simulink model "ieee30"  (R2017a)
settings: Solver=VariableStepDiscrete  StartTime=0.0  StopTime=0.012  MaxStep=1e-4  RelTol=1e-3
undefined symbols (not defined in the file): Angle, Magnitude
libraries: powerlib x548
(part 4 of 4)

== system ieee30/Line 16-17-2 ==
  Line{,1..4} (5 alike) : powerlib/Elements/Three-Phase PI Section Line  LConnTagsString=a|b|c  RConnTagsString=A|B|C  Frequency=60  Resistances=[rt ro] /100  Inductances=[ lt lo] /100  Capacitances=[ct co]/100  Length=20
      settings: SourceProductName=Simscape Power Systems
  A : PMIOPort  Port=1  Side=Left
  B : PMIOPort  Port=2  Side=Left
  C : PMIOPort  Port=3  Side=Left
  a : PMIOPort  Port=4  Side=Right
  b : PMIOPort  Port=5  Side=Right
  c : PMIOPort  Port=6  Side=Right
  connections:
  Line3/RConn3 -- Line4/LConn3
  Line/RConn3 -- Line1/LConn3
  Line2/RConn3 -- Line3/LConn3
  Line2/RConn1 -- Line3/LConn1
  Line1/RConn3 -- Line2/LConn3
  Line/RConn2 -- Line1/LConn2
  Line2/RConn2 -- Line3/LConn2
  Line1/RConn1 -- Line2/LConn1
  Line3/RConn1 -- Line4/LConn1
  Line3/RConn2 -- Line4/LConn2
  Line1/RConn2 -- Line2/LConn2
  Line/RConn1 -- Line1/LConn1
  C/RConn1 -- Line/LConn3
  Line/LConn1 -- A/RConn1
  c/RConn1 -- Line4/RConn3
  a/RConn1 -- Line4/RConn1
  B/RConn1 -- Line/LConn2
  b/RConn1 -- Line4/RConn2

== system ieee30/Line 18-19-1 ==
  Line{,1..4} (5 alike) : powerlib/Elements/Three-Phase PI Section Line  LConnTagsString=a|b|c  RConnTagsString=A|B|C  Frequency=60  Resistances=[rt ro] /100  Inductances=[ lt lo] /100  Capacitances=[ct co]/100  Length=20
      settings: SourceProductName=Simscape Power Systems
  A : PMIOPort  Port=1  Side=Left
  B : PMIOPort  Port=2  Side=Left
  C : PMIOPort  Port=3  Side=Left
  a : PMIOPort  Port=4  Side=Right
  b : PMIOPort  Port=5  Side=Right
  c : PMIOPort  Port=6  Side=Right
  connections:
  Line3/RConn3 -- Line4/LConn3
  Line/RConn3 -- Line1/LConn3
  Line2/RConn3 -- Line3/LConn3
  Line2/RConn1 -- Line3/LConn1
  Line1/RConn3 -- Line2/LConn3
  Line/RConn2 -- Line1/LConn2
  Line2/RConn2 -- Line3/LConn2
  Line1/RConn1 -- Line2/LConn1
  Line3/RConn1 -- Line4/LConn1
  Line3/RConn2 -- Line4/LConn2
  Line1/RConn2 -- Line2/LConn2
  Line/RConn1 -- Line1/LConn1
  C/RConn1 -- Line/LConn3
  Line/LConn1 -- A/RConn1
  c/RConn1 -- Line4/RConn3
  a/RConn1 -- Line4/RConn1
  B/RConn1 -- Line/LConn2
  b/RConn1 -- Line4/RConn2

== system ieee30/Line 18-19-2 ==
  Line{,1..4} (5 alike) : powerlib/Elements/Three-Phase PI Section Line  LConnTagsString=a|b|c  RConnTagsString=A|B|C  Frequency=60  Resistances=[rt ro] /100  Inductances=[ lt lo] /100  Capacitances=[ct co]/100  Length=20
      settings: SourceProductName=Simscape Power Systems
  A : PMIOPort  Port=1  Side=Left
  B : PMIOPort  Port=2  Side=Left
  C : PMIOPort  Port=3  Side=Left
  a : PMIOPort  Port=4  Side=Right
  b : PMIOPort  Port=5  Side=Right
  c : PMIOPort  Port=6  Side=Right
  connections:
  Line3/RConn3 -- Line4/LConn3
  Line/RConn3 -- Line1/LConn3
  Line2/RConn3 -- Line3/LConn3
  Line2/RConn1 -- Line3/LConn1
  Line1/RConn3 -- Line2/LConn3
  Line/RConn2 -- Line1/LConn2
  Line2/RConn2 -- Line3/LConn2
  Line1/RConn1 -- Line2/LConn1
  Line3/RConn1 -- Line4/LConn1
  Line3/RConn2 -- Line4/LConn2
  Line1/RConn2 -- Line2/LConn2
  Line/RConn1 -- Line1/LConn1
  C/RConn1 -- Line/LConn3
  Line/LConn1 -- A/RConn1
  c/RConn1 -- Line4/RConn3
  a/RConn1 -- Line4/RConn1
  B/RConn1 -- Line/LConn2
  b/RConn1 -- Line4/RConn2

== system ieee30/Line 19-20-1 ==
  Line{,1..4} (5 alike) : powerlib/Elements/Three-Phase PI Section Line  LConnTagsString=a|b|c  RConnTagsString=A|B|C  Frequency=60  Resistances=[rt ro] /100  Inductances=[ lt lo] /100  Capacitances=[ct co]/100  Length=20
      settings: SourceProductName=Simscape Power Systems
  A : PMIOPort  Port=1  Side=Left
  B : PMIOPort  Port=2  Side=Left
  C : PMIOPort  Port=3  Side=Left
  a : PMIOPort  Port=4  Side=Right
  b : PMIOPort  Port=5  Side=Right
  c : PMIOPort  Port=6  Side=Right
  connections:
  Line3/RConn3 -- Line4/LConn3
  Line/RConn3 -- Line1/LConn3
  Line2/RConn3 -- Line3/LConn3
  Line2/RConn1 -- Line3/LConn1
  Line1/RConn3 -- Line2/LConn3
  Line/RConn2 -- Line1/LConn2
  Line2/RConn2 -- Line3/LConn2
  Line1/RConn1 -- Line2/LConn1
  Line3/RConn1 -- Line4/LConn1
  Line3/RConn2 -- Line4/LConn2
  Line1/RConn2 -- Line2/LConn2
  Line/RConn1 -- Line1/LConn1
  C/RConn1 -- Line/LConn3
  Line/LConn1 -- A/RConn1
  c/RConn1 -- Line4/RConn3
  a/RConn1 -- Line4/RConn1
  B/RConn1 -- Line/LConn2
  b/RConn1 -- Line4/RConn2

== system ieee30/Line 19-20-2 ==
  Line{,1..4} (5 alike) : powerlib/Elements/Three-Phase PI Section Line  LConnTagsString=a|b|c  RConnTagsString=A|B|C  Frequency=60  Resistances=[rt ro] /100  Inductances=[ lt lo] /100  Capacitances=[ct co]/100  Length=20
      settings: SourceProductName=Simscape Power Systems
  A : PMIOPort  Port=1  Side=Left
  B : PMIOPort  Port=2  Side=Left
  C : PMIOPort  Port=3  Side=Left
  a : PMIOPort  Port=4  Side=Right
  b : PMIOPort  Port=5  Side=Right
  c : PMIOPort  Port=6  Side=Right
  connections:
  Line3/RConn3 -- Line4/LConn3
  Line/RConn3 -- Line1/LConn3
  Line2/RConn3 -- Line3/LConn3
  Line2/RConn1 -- Line3/LConn1
  Line1/RConn3 -- Line2/LConn3
  Line/RConn2 -- Line1/LConn2
  Line2/RConn2 -- Line3/LConn2
  Line1/RConn1 -- Line2/LConn1
  Line3/RConn1 -- Line4/LConn1
  Line3/RConn2 -- Line4/LConn2
  Line1/RConn2 -- Line2/LConn2
  Line/RConn1 -- Line1/LConn1
  C/RConn1 -- Line/LConn3
  Line/LConn1 -- A/RConn1
  c/RConn1 -- Line4/RConn3
  a/RConn1 -- Line4/RConn1
  B/RConn1 -- Line/LConn2
  b/RConn1 -- Line4/RConn2

== system ieee30/Line 2-4-1 ==
  Line{,1..4} (5 alike) : powerlib/Elements/Three-Phase PI Section Line  LConnTagsString=a|b|c  RConnTagsString=A|B|C  Frequency=60  Resistances=[rt ro] /100  Inductances=[ lt lo] /100  Capacitances=[ct co]/100  Length=20
      settings: SourceProductName=Simscape Power Systems
  A : PMIOPort  Port=1  Side=Left
  B : PMIOPort  Port=2  Side=Left
  C : PMIOPort  Port=3  Side=Left
  a : PMIOPort  Port=4  Side=Right
  b : PMIOPort  Port=5  Side=Right
  c : PMIOPort  Port=6  Side=Right
  connections:
  Line3/RConn3 -- Line4/LConn3
  Line/RConn3 -- Line1/LConn3
  Line2/RConn3 -- Line3/LConn3
  Line2/RConn1 -- Line3/LConn1
  Line1/RConn3 -- Line2/LConn3
  Line/RConn2 -- Line1/LConn2
  Line2/RConn2 -- Line3/LConn2
  Line1/RConn1 -- Line2/LConn1
  Line3/RConn1 -- Line4/LConn1
  Line3/RConn2 -- Line4/LConn2
  Line1/RConn2 -- Line2/LConn2
  Line/RConn1 -- Line1/LConn1
  C/RConn1 -- Line/LConn3
  Line/LConn1 -- A/RConn1
  c/RConn1 -- Line4/RConn3
  a/RConn1 -- Line4/RConn1
  B/RConn1 -- Line/LConn2
  b/RConn1 -- Line4/RConn2

== system ieee30/Line 2-4-2 ==
  Line{,1..4} (5 alike) : powerlib/Elements/Three-Phase PI Section Line  LConnTagsString=a|b|c  RConnTagsString=A|B|C  Frequency=60  Resistances=[rt ro] /100  Inductances=[ lt lo] /100  Capacitances=[ct co]/100  Length=20
      settings: SourceProductName=Simscape Power Systems
  A : PMIOPort  Port=1  Side=Left
  B : PMIOPort  Port=2  Side=Left
  C : PMIOPort  Port=3  Side=Left
  a : PMIOPort  Port=4  Side=Right
  b : PMIOPort  Port=5  Side=Right
  c : PMIOPort  Port=6  Side=Right
  connections:
  Line3/RConn3 -- Line4/LConn3
  Line/RConn3 -- Line1/LConn3
  Line2/RConn3 -- Line3/LConn3
  Line2/RConn1 -- Line3/LConn1
  Line1/RConn3 -- Line2/LConn3
  Line/RConn2 -- Line1/LConn2
  Line2/RConn2 -- Line3/LConn2
  Line1/RConn1 -- Line2/LConn1
  Line3/RConn1 -- Line4/LConn1
  Line3/RConn2 -- Line4/LConn2
  Line1/RConn2 -- Line2/LConn2
  Line/RConn1 -- Line1/LConn1
  C/RConn1 -- Line/LConn3
  Line/LConn1 -- A/RConn1
  c/RConn1 -- Line4/RConn3
  a/RConn1 -- Line4/RConn1
  B/RConn1 -- Line/LConn2
  b/RConn1 -- Line4/RConn2

== system ieee30/Line 2-5-1 ==
  Line{,1..4} (5 alike) : powerlib/Elements/Three-Phase PI Section Line  LConnTagsString=a|b|c  RConnTagsString=A|B|C  Frequency=60  Resistances=[rt ro] /100  Inductances=[ lt lo] /100  Capacitances=[ct co]/100  Length=20
      settings: SourceProductName=Simscape Power Systems
  A : PMIOPort  Port=1  Side=Left
  B : PMIOPort  Port=2  Side=Left
  C : PMIOPort  Port=3  Side=Left
  a : PMIOPort  Port=4  Side=Right
  b : PMIOPort  Port=5  Side=Right
  c : PMIOPort  Port=6  Side=Right
  connections:
  Line3/RConn3 -- Line4/LConn3
  Line/RConn3 -- Line1/LConn3
  Line2/RConn3 -- Line3/LConn3
  Line2/RConn1 -- Line3/LConn1
  Line1/RConn3 -- Line2/LConn3
  Line/RConn2 -- Line1/LConn2
  Line2/RConn2 -- Line3/LConn2
  Line1/RConn1 -- Line2/LConn1
  Line3/RConn1 -- Line4/LConn1
  Line3/RConn2 -- Line4/LConn2
  Line1/RConn2 -- Line2/LConn2
  Line/RConn1 -- Line1/LConn1
  C/RConn1 -- Line/LConn3
  Line/LConn1 -- A/RConn1
  c/RConn1 -- Line4/RConn3
  a/RConn1 -- Line4/RConn1
  B/RConn1 -- Line/LConn2
  b/RConn1 -- Line4/RConn2

== system ieee30/Line 2-5-2 ==
  Line{,1..4} (5 alike) : powerlib/Elements/Three-Phase PI Section Line  LConnTagsString=a|b|c  RConnTagsString=A|B|C  Frequency=60  Resistances=[rt ro] /100  Inductances=[ lt lo] /100  Capacitances=[ct co]/100  Length=20
      settings: SourceProductName=Simscape Power Systems
  A : PMIOPort  Port=1  Side=Left
  B : PMIOPort  Port=2  Side=Left
  C : PMIOPort  Port=3  Side=Left
  a : PMIOPort  Port=4  Side=Right
  b : PMIOPort  Port=5  Side=Right
  c : PMIOPort  Port=6  Side=Right
  connections:
  Line3/RConn3 -- Line4/LConn3
  Line/RConn3 -- Line1/LConn3
  Line2/RConn3 -- Line3/LConn3
  Line2/RConn1 -- Line3/LConn1
  Line1/RConn3 -- Line2/LConn3
  Line/RConn2 -- Line1/LConn2
  Line2/RConn2 -- Line3/LConn2
  Line1/RConn1 -- Line2/LConn1
  Line3/RConn1 -- Line4/LConn1
  Line3/RConn2 -- Line4/LConn2
  Line1/RConn2 -- Line2/LConn2
  Line/RConn1 -- Line1/LConn1
  C/RConn1 -- Line/LConn3
  Line/LConn1 -- A/RConn1
  c/RConn1 -- Line4/RConn3
  a/RConn1 -- Line4/RConn1
  B/RConn1 -- Line/LConn2
  b/RConn1 -- Line4/RConn2

== system ieee30/Line 2-6-1 ==
  Line{,1..4} (5 alike) : powerlib/Elements/Three-Phase PI Section Line  LConnTagsString=a|b|c  RConnTagsString=A|B|C  Frequency=60  Resistances=[rt ro] /100  Inductances=[ lt lo] /100  Capacitances=[ct co]/100  Length=20
      settings: SourceProductName=Simscape Power Systems
  A : PMIOPort  Port=1  Side=Left
  B : PMIOPort  Port=2  Side=Left
  C : PMIOPort  Port=3  Side=Left
  a : PMIOPort  Port=4  Side=Right
  b : PMIOPort  Port=5  Side=Right
  c : PMIOPort  Port=6  Side=Right
  connections:
  Line3/RConn3 -- Line4/LConn3
  Line/RConn3 -- Line1/LConn3
  Line2/RConn3 -- Line3/LConn3
  Line2/RConn1 -- Line3/LConn1
  Line1/RConn3 -- Line2/LConn3
  Line/RConn2 -- Line1/LConn2
  Line2/RConn2 -- Line3/LConn2
  Line1/RConn1 -- Line2/LConn1
  Line3/RConn1 -- Line4/LConn1
  Line3/RConn2 -- Line4/LConn2
  Line1/RConn2 -- Line2/LConn2
  Line/RConn1 -- Line1/LConn1
  C/RConn1 -- Line/LConn3
  Line/LConn1 -- A/RConn1
  c/RConn1 -- Line4/RConn3
  a/RConn1 -- Line4/RConn1
  B/RConn1 -- Line/LConn2
  b/RConn1 -- Line4/RConn2

== system ieee30/Line 2-6-2 ==
  Line{,1..4} (5 alike) : powerlib/Elements/Three-Phase PI Section Line  LConnTagsString=a|b|c  RConnTagsString=A|B|C  Frequency=60  Resistances=[rt ro] /100  Inductances=[ lt lo] /100  Capacitances=[ct co]/100  Length=20
      settings: SourceProductName=Simscape Power Systems
  A : PMIOPort  Port=1  Side=Left
  B : PMIOPort  Port=2  Side=Left
  C : PMIOPort  Port=3  Side=Left
  a : PMIOPort  Port=4  Side=Right
  b : PMIOPort  Port=5  Side=Right
  c : PMIOPort  Port=6  Side=Right
  connections:
  Line3/RConn3 -- Line4/LConn3
  Line/RConn3 -- Line1/LConn3
  Line2/RConn3 -- Line3/LConn3
  Line2/RConn1 -- Line3/LConn1
  Line1/RConn3 -- Line2/LConn3
  Line/RConn2 -- Line1/LConn2
  Line2/RConn2 -- Line3/LConn2
  Line1/RConn1 -- Line2/LConn1
  Line3/RConn1 -- Line4/LConn1
  Line3/RConn2 -- Line4/LConn2
  Line1/RConn2 -- Line2/LConn2
  Line/RConn1 -- Line1/LConn1
  C/RConn1 -- Line/LConn3
  Line/LConn1 -- A/RConn1
  c/RConn1 -- Line4/RConn3
  a/RConn1 -- Line4/RConn1
  B/RConn1 -- Line/LConn2
  b/RConn1 -- Line4/RConn2

== system ieee30/Line 21-22-1 ==
  Line{,1..4} (5 alike) : powerlib/Elements/Three-Phase PI Section Line  LConnTagsString=a|b|c  RConnTagsString=A|B|C  Frequency=60  Resistances=[rt ro] /100  Inductances=[ lt lo] /100  Capacitances=[ct co]/100  Length=20
      settings: SourceProductName=Simscape Power Systems
  A : PMIOPort  Port=1  Side=Left
  B : PMIOPort  Port=2  Side=Left
  C : PMIOPort  Port=3  Side=Left
  a : PMIOPort  Port=4  Side=Right
  b : PMIOPort  Port=5  Side=Right
  c : PMIOPort  Port=6  Side=Right
  connections:
  Line3/RConn3 -- Line4/LConn3
  Line/RConn3 -- Line1/LConn3
  Line2/RConn3 -- Line3/LConn3
  Line2/RConn1 -- Line3/LConn1
  Line1/RConn3 -- Line2/LConn3
  Line/RConn2 -- Line1/LConn2
  Line2/RConn2 -- Line3/LConn2
  Line1/RConn1 -- Line2/LConn1
  Line3/RConn1 -- Line4/LConn1
  Line3/RConn2 -- Line4/LConn2
  Line1/RConn2 -- Line2/LConn2
  Line/RConn1 -- Line1/LConn1
  C/RConn1 -- Line/LConn3
  Line/LConn1 -- A/RConn1
  c/RConn1 -- Line4/RConn3
  a/RConn1 -- Line4/RConn1
  B/RConn1 -- Line/LConn2
  b/RConn1 -- Line4/RConn2

== system ieee30/Line 21-22-2 ==
  Line{,1..4} (5 alike) : powerlib/Elements/Three-Phase PI Section Line  LConnTagsString=a|b|c  RConnTagsString=A|B|C  Frequency=60  Resistances=[rt ro] /100  Inductances=[ lt lo] /100  Capacitances=[ct co]/100  Length=20
      settings: SourceProductName=Simscape Power Systems
  A : PMIOPort  Port=1  Side=Left
  B : PMIOPort  Port=2  Side=Left
  C : PMIOPort  Port=3  Side=Left
  a : PMIOPort  Port=4  Side=Right
  b : PMIOPort  Port=5  Side=Right
  c : PMIOPort  Port=6  Side=Right
  connections:
  Line3/RConn3 -- Line4/LConn3
  Line/RConn3 -- Line1/LConn3
  Line2/RConn3 -- Line3/LConn3
  Line2/RConn1 -- Line3/LConn1
  Line1/RConn3 -- Line2/LConn3
  Line/RConn2 -- Line1/LConn2
  Line2/RConn2 -- Line3/LConn2
  Line1/RConn1 -- Line2/LConn1
  Line3/RConn1 -- Line4/LConn1
  Line3/RConn2 -- Line4/LConn2
  Line1/RConn2 -- Line2/LConn2
  Line/RConn1 -- Line1/LConn1
  C/RConn1 -- Line/LConn3
  Line/LConn1 -- A/RConn1
  c/RConn1 -- Line4/RConn3
  a/RConn1 -- Line4/RConn1
  B/RConn1 -- Line/LConn2
  b/RConn1 -- Line4/RConn2

== system ieee30/Line 22-24-1 ==
  Line{,1..4} (5 alike) : powerlib/Elements/Three-Phase PI Section Line  LConnTagsString=a|b|c  RConnTagsString=A|B|C  Frequency=60  Resistances=[rt ro] /100  Inductances=[ lt lo] /100  Capacitances=[ct co]/100  Length=20
      settings: SourceProductName=Simscape Power Systems
  A : PMIOPort  Port=1  Side=Left
  B : PMIOPort  Port=2  Side=Left
  C : PMIOPort  Port=3  Side=Left
  a : PMIOPort  Port=4  Side=Right
  b : PMIOPort  Port=5  Side=Right
  c : PMIOPort  Port=6  Side=Right
  connections:
  Line3/RConn3 -- Line4/LConn3
  Line/RConn3 -- Line1/LConn3
  Line2/RConn3 -- Line3/LConn3
  Line2/RConn1 -- Line3/LConn1
  Line1/RConn3 -- Line2/LConn3
  Line/RConn2 -- Line1/LConn2
  Line2/RConn2 -- Line3/LConn2
  Line1/RConn1 -- Line2/LConn1
  Line3/RConn1 -- Line4/LConn1
  Line3/RConn2 -- Line4/LConn2
  Line1/RConn2 -- Line2/LConn2
  Line/RConn1 -- Line1/LConn1
  C/RConn1 -- Line/LConn3
  Line/LConn1 -- A/RConn1
  c/RConn1 -- Line4/RConn3
  a/RConn1 -- Line4/RConn1
  B/RConn1 -- Line/LConn2
  b/RConn1 -- Line4/RConn2

== system ieee30/Line 22-24-2 ==
  Line{,1..4} (5 alike) : powerlib/Elements/Three-Phase PI Section Line  LConnTagsString=a|b|c  RConnTagsString=A|B|C  Frequency=60  Resistances=[rt ro] /100  Inductances=[ lt lo] /100  Capacitances=[ct co]/100  Length=20
      settings: SourceProductName=Simscape Power Systems
  A : PMIOPort  Port=1  Side=Left
  B : PMIOPort  Port=2  Side=Left
  C : PMIOPort  Port=3  Side=Left
  a : PMIOPort  Port=4  Side=Right
  b : PMIOPort  Port=5  Side=Right
  c : PMIOPort  Port=6  Side=Right
  connections:
  Line3/RConn3 -- Line4/LConn3
  Line/RConn3 -- Line1/LConn3
  Line2/RConn3 -- Line3/LConn3
  Line2/RConn1 -- Line3/LConn1
  Line1/RConn3 -- Line2/LConn3
  Line/RConn2 -- Line1/LConn2
  Line2/RConn2 -- Line3/LConn2
  Line1/RConn1 -- Line2/LConn1
  Line3/RConn1 -- Line4/LConn1
  Line3/RConn2 -- Line4/LConn2
  Line1/RConn2 -- Line2/LConn2
  Line/RConn1 -- Line1/LConn1
  C/RConn1 -- Line/LConn3
  Line/LConn1 -- A/RConn1
  c/RConn1 -- Line4/RConn3
  a/RConn1 -- Line4/RConn1
  B/RConn1 -- Line/LConn2
  b/RConn1 -- Line4/RConn2

== system ieee30/Line 23-24-1 ==
  Line{,1..4} (5 alike) : powerlib/Elements/Three-Phase PI Section Line  LConnTagsString=a|b|c  RConnTagsString=A|B|C  Frequency=60  Resistances=[rt ro] /100  Inductances=[ lt lo] /100  Capacitances=[ct co]/100  Length=20
      settings: SourceProductName=Simscape Power Systems
  A : PMIOPort  Port=1  Side=Left
  B : PMIOPort  Port=2  Side=Left
  C : PMIOPort  Port=3  Side=Left
  a : PMIOPort  Port=4  Side=Right
  b : PMIOPort  Port=5  Side=Right
  c : PMIOPort  Port=6  Side=Right
  connections:
  Line3/RConn3 -- Line4/LConn3
  Line/RConn3 -- Line1/LConn3
  Line2/RConn3 -- Line3/LConn3
  Line2/RConn1 -- Line3/LConn1
  Line1/RConn3 -- Line2/LConn3
  Line/RConn2 -- Line1/LConn2
  Line2/RConn2 -- Line3/LConn2
  Line1/RConn1 -- Line2/LConn1
  Line3/RConn1 -- Line4/LConn1
  Line3/RConn2 -- Line4/LConn2
  Line1/RConn2 -- Line2/LConn2
  Line/RConn1 -- Line1/LConn1
  C/RConn1 -- Line/LConn3
  Line/LConn1 -- A/RConn1
  c/RConn1 -- Line4/RConn3
  a/RConn1 -- Line4/RConn1
  B/RConn1 -- Line/LConn2
  b/RConn1 -- Line4/RConn2

== system ieee30/Line 23-24-2 ==
  Line{,1..4} (5 alike) : powerlib/Elements/Three-Phase PI Section Line  LConnTagsString=a|b|c  RConnTagsString=A|B|C  Frequency=60  Resistances=[rt ro] /100  Inductances=[ lt lo] /100  Capacitances=[ct co]/100  Length=20
      settings: SourceProductName=Simscape Power Systems
  A : PMIOPort  Port=1  Side=Left
  B : PMIOPort  Port=2  Side=Left
  C : PMIOPort  Port=3  Side=Left
  a : PMIOPort  Port=4  Side=Right
  b : PMIOPort  Port=5  Side=Right
  c : PMIOPort  Port=6  Side=Right
  connections:
  Line3/RConn3 -- Line4/LConn3
  Line/RConn3 -- Line1/LConn3
  Line2/RConn3 -- Line3/LConn3
  Line2/RConn1 -- Line3/LConn1
  Line1/RConn3 -- Line2/LConn3
  Line/RConn2 -- Line1/LConn2
  Line2/RConn2 -- Line3/LConn2
  Line1/RConn1 -- Line2/LConn1
  Line3/RConn1 -- Line4/LConn1
  Line3/RConn2 -- Line4/LConn2
  Line1/RConn2 -- Line2/LConn2
  Line/RConn1 -- Line1/LConn1
  C/RConn1 -- Line/LConn3
  Line/LConn1 -- A/RConn1
  c/RConn1 -- Line4/RConn3
  a/RConn1 -- Line4/RConn1
  B/RConn1 -- Line/LConn2
  b/RConn1 -- Line4/RConn2

== system ieee30/Line 24-25-1 ==
  Line{,1..4} (5 alike) : powerlib/Elements/Three-Phase PI Section Line  LConnTagsString=a|b|c  RConnTagsString=A|B|C  Frequency=60  Resistances=[rt ro] /100  Inductances=[ lt lo] /100  Capacitances=[ct co]/100  Length=20
      settings: SourceProductName=Simscape Power Systems
  A : PMIOPort  Port=1  Side=Left
  B : PMIOPort  Port=2  Side=Left
  C : PMIOPort  Port=3  Side=Left
  a : PMIOPort  Port=4  Side=Right
  b : PMIOPort  Port=5  Side=Right
  c : PMIOPort  Port=6  Side=Right
  connections:
  Line3/RConn3 -- Line4/LConn3
  Line/RConn3 -- Line1/LConn3
  Line2/RConn3 -- Line3/LConn3
  Line2/RConn1 -- Line3/LConn1
  Line1/RConn3 -- Line2/LConn3
  Line/RConn2 -- Line1/LConn2
  Line2/RConn2 -- Line3/LConn2
  Line1/RConn1 -- Line2/LConn1
  Line3/RConn1 -- Line4/LConn1
  Line3/RConn2 -- Line4/LConn2
  Line1/RConn2 -- Line2/LConn2
  Line/RConn1 -- Line1/LConn1
  C/RConn1 -- Line/LConn3
  Line/LConn1 -- A/RConn1
  c/RConn1 -- Line4/RConn3
  a/RConn1 -- Line4/RConn1
  B/RConn1 -- Line/LConn2
  b/RConn1 -- Line4/RConn2

== system ieee30/Line 24-25-2 ==
  Line{,1..4} (5 alike) : powerlib/Elements/Three-Phase PI Section Line  LConnTagsString=a|b|c  RConnTagsString=A|B|C  Frequency=60  Resistances=[rt ro] /100  Inductances=[ lt lo] /100  Capacitances=[ct co]/100  Length=20
      settings: SourceProductName=Simscape Power Systems
  A : PMIOPort  Port=1  Side=Left
  B : PMIOPort  Port=2  Side=Left
  C : PMIOPort  Port=3  Side=Left
  a : PMIOPort  Port=4  Side=Right
  b : PMIOPort  Port=5  Side=Right
  c : PMIOPort  Port=6  Side=Right
  connections:
  Line3/RConn3 -- Line4/LConn3
  Line/RConn3 -- Line1/LConn3
  Line2/RConn3 -- Line3/LConn3
  Line2/RConn1 -- Line3/LConn1
  Line1/RConn3 -- Line2/LConn3
  Line/RConn2 -- Line1/LConn2
  Line2/RConn2 -- Line3/LConn2
  Line1/RConn1 -- Line2/LConn1
  Line3/RConn1 -- Line4/LConn1
  Line3/RConn2 -- Line4/LConn2
  Line1/RConn2 -- Line2/LConn2
  Line/RConn1 -- Line1/LConn1
  C/RConn1 -- Line/LConn3
  Line/LConn1 -- A/RConn1
  c/RConn1 -- Line4/RConn3
  a/RConn1 -- Line4/RConn1
  B/RConn1 -- Line/LConn2
  b/RConn1 -- Line4/RConn2

== system ieee30/Line 25-26-1 ==
  Line{,1..4} (5 alike) : powerlib/Elements/Three-Phase PI Section Line  LConnTagsString=a|b|c  RConnTagsString=A|B|C  Frequency=60  Resistances=[rt ro] /100  Inductances=[ lt lo] /100  Capacitances=[ct co]/100  Length=20
      settings: SourceProductName=Simscape Power Systems
  A : PMIOPort  Port=1  Side=Left
  B : PMIOPort  Port=2  Side=Left
  C : PMIOPort  Port=3  Side=Left
  a : PMIOPort  Port=4  Side=Right
  b : PMIOPort  Port=5  Side=Right
  c : PMIOPort  Port=6  Side=Right
  connections:
  Line3/RConn3 -- Line4/LConn3
  Line/RConn3 -- Line1/LConn3
  Line2/RConn3 -- Line3/LConn3
  Line2/RConn1 -- Line3/LConn1
  Line1/RConn3 -- Line2/LConn3
  Line/RConn2 -- Line1/LConn2
  Line2/RConn2 -- Line3/LConn2
  Line1/RConn1 -- Line2/LConn1
  Line3/RConn1 -- Line4/LConn1
  Line3/RConn2 -- Line4/LConn2
  Line1/RConn2 -- Line2/LConn2
  Line/RConn1 -- Line1/LConn1
  C/RConn1 -- Line/LConn3
  Line/LConn1 -- A/RConn1
  c/RConn1 -- Line4/RConn3
  a/RConn1 -- Line4/RConn1
  B/RConn1 -- Line/LConn2
  b/RConn1 -- Line4/RConn2

== system ieee30/Line 25-26-2 ==
  Line{,1..4} (5 alike) : powerlib/Elements/Three-Phase PI Section Line  LConnTagsString=a|b|c  RConnTagsString=A|B|C  Frequency=60  Resistances=[rt ro] /100  Inductances=[ lt lo] /100  Capacitances=[ct co]/100  Length=20
      settings: SourceProductName=Simscape Power Systems
  A : PMIOPort  Port=1  Side=Left
  B : PMIOPort  Port=2  Side=Left
  C : PMIOPort  Port=3  Side=Left
  a : PMIOPort  Port=4  Side=Right
  b : PMIOPort  Port=5  Side=Right
  c : PMIOPort  Port=6  Side=Right
  connections:
  Line3/RConn3 -- Line4/LConn3
  Line/RConn3 -- Line1/LConn3
  Line2/RConn3 -- Line3/LConn3
  Line2/RConn1 -- Line3/LConn1
  Line1/RConn3 -- Line2/LConn3
  Line/RConn2 -- Line1/LConn2
  Line2/RConn2 -- Line3/LConn2
  Line1/RConn1 -- Line2/LConn1
  Line3/RConn1 -- Line4/LConn1
  Line3/RConn2 -- Line4/LConn2
  Line1/RConn2 -- Line2/LConn2
  Line/RConn1 -- Line1/LConn1
  C/RConn1 -- Line/LConn3
  Line/LConn1 -- A/RConn1
  c/RConn1 -- Line4/RConn3
  a/RConn1 -- Line4/RConn1
  B/RConn1 -- Line/LConn2
  b/RConn1 -- Line4/RConn2

== system ieee30/Line 25-27-1 ==
  Line{,1..4} (5 alike) : powerlib/Elements/Three-Phase PI Section Line  LConnTagsString=a|b|c  RConnTagsString=A|B|C  Frequency=60  Resistances=[rt ro] /100  Inductances=[ lt lo] /100  Capacitances=[ct co]/100  Length=20
      settings: SourceProductName=Simscape Power Systems
  A : PMIOPort  Port=1  Side=Left
  B : PMIOPort  Port=2  Side=Left
  C : PMIOPort  Port=3  Side=Left
  a : PMIOPort  Port=4  Side=Right
  b : PMIOPort  Port=5  Side=Right
  c : PMIOPort  Port=6  Side=Right
  connections:
  Line3/RConn3 -- Line4/LConn3
  Line/RConn3 -- Line1/LConn3
  Line2/RConn3 -- Line3/LConn3
  Line2/RConn1 -- Line3/LConn1
  Line1/RConn3 -- Line2/LConn3
  Line/RConn2 -- Line1/LConn2
  Line2/RConn2 -- Line3/LConn2
  Line1/RConn1 -- Line2/LConn1
  Line3/RConn1 -- Line4/LConn1
  Line3/RConn2 -- Line4/LConn2
  Line1/RConn2 -- Line2/LConn2
  Line/RConn1 -- Line1/LConn1
  C/RConn1 -- Line/LConn3
  Line/LConn1 -- A/RConn1
  c/RConn1 -- Line4/RConn3
  a/RConn1 -- Line4/RConn1
  B/RConn1 -- Line/LConn2
  b/RConn1 -- Line4/RConn2

== system ieee30/Line 25-27-2 ==
  Line{,1..4} (5 alike) : powerlib/Elements/Three-Phase PI Section Line  LConnTagsString=a|b|c  RConnTagsString=A|B|C  Frequency=60  Resistances=[rt ro] /100  Inductances=[ lt lo] /100  Capacitances=[ct co]/100  Length=20
      settings: SourceProductName=Simscape Power Systems
  A : PMIOPort  Port=1  Side=Left
  B : PMIOPort  Port=2  Side=Left
  C : PMIOPort  Port=3  Side=Left
  a : PMIOPort  Port=4  Side=Right
  b : PMIOPort  Port=5  Side=Right
  c : PMIOPort  Port=6  Side=Right
  connections:
  Line3/RConn3 -- Line4/LConn3
  Line/RConn3 -- Line1/LConn3
  Line2/RConn3 -- Line3/LConn3
  Line2/RConn1 -- Line3/LConn1
  Line1/RConn3 -- Line2/LConn3
  Line/RConn2 -- Line1/LConn2
  Line2/RConn2 -- Line3/LConn2
  Line1/RConn1 -- Line2/LConn1
  Line3/RConn1 -- Line4/LConn1
  Line3/RConn2 -- Line4/LConn2
  Line1/RConn2 -- Line2/LConn2
  Line/RConn1 -- Line1/LConn1
  C/RConn1 -- Line/LConn3
  Line/LConn1 -- A/RConn1
  c/RConn1 -- Line4/RConn3
  a/RConn1 -- Line4/RConn1
  B/RConn1 -- Line/LConn2
  b/RConn1 -- Line4/RConn2

== system ieee30/Line 27-29-1 ==
  Line{,1..4} (5 alike) : powerlib/Elements/Three-Phase PI Section Line  LConnTagsString=a|b|c  RConnTagsString=A|B|C  Frequency=60  Resistances=[rt ro] /100  Inductances=[ lt lo] /100  Capacitances=[ct co]/100  Length=20
      settings: SourceProductName=Simscape Power Systems
  A : PMIOPort  Port=1  Side=Left
  B : PMIOPort  Port=2  Side=Left
  C : PMIOPort  Port=3  Side=Left
  a : PMIOPort  Port=4  Side=Right
  b : PMIOPort  Port=5  Side=Right
  c : PMIOPort  Port=6  Side=Right
  connections:
  Line3/RConn3 -- Line4/LConn3
  Line/RConn3 -- Line1/LConn3
  Line2/RConn3 -- Line3/LConn3
  Line2/RConn1 -- Line3/LConn1
  Line1/RConn3 -- Line2/LConn3
  Line/RConn2 -- Line1/LConn2
  Line2/RConn2 -- Line3/LConn2
  Line1/RConn1 -- Line2/LConn1
  Line3/RConn1 -- Line4/LConn1
  Line3/RConn2 -- Line4/LConn2
  Line1/RConn2 -- Line2/LConn2
  Line/RConn1 -- Line1/LConn1
  C/RConn1 -- Line/LConn3
  Line/LConn1 -- A/RConn1
  c/RConn1 -- Line4/RConn3
  a/RConn1 -- Line4/RConn1
  B/RConn1 -- Line/LConn2
  b/RConn1 -- Line4/RConn2

== system ieee30/Line 27-29-2 ==
  Line{,1..4} (5 alike) : powerlib/Elements/Three-Phase PI Section Line  LConnTagsString=a|b|c  RConnTagsString=A|B|C  Frequency=60  Resistances=[rt ro] /100  Inductances=[ lt lo] /100  Capacitances=[ct co]/100  Length=20
      settings: SourceProductName=Simscape Power Systems
  A : PMIOPort  Port=1  Side=Left
  B : PMIOPort  Port=2  Side=Left
  C : PMIOPort  Port=3  Side=Left
  a : PMIOPort  Port=4  Side=Right
  b : PMIOPort  Port=5  Side=Right
  c : PMIOPort  Port=6  Side=Right
  connections:
  Line3/RConn3 -- Line4/LConn3
  Line/RConn3 -- Line1/LConn3
  Line2/RConn3 -- Line3/LConn3
  Line2/RConn1 -- Line3/LConn1
  Line1/RConn3 -- Line2/LConn3
  Line/RConn2 -- Line1/LConn2
  Line2/RConn2 -- Line3/LConn2
  Line1/RConn1 -- Line2/LConn1
  Line3/RConn1 -- Line4/LConn1
  Line3/RConn2 -- Line4/LConn2
  Line1/RConn2 -- Line2/LConn2
  Line/RConn1 -- Line1/LConn1
  C/RConn1 -- Line/LConn3
  Line/LConn1 -- A/RConn1
  c/RConn1 -- Line4/RConn3
  a/RConn1 -- Line4/RConn1
  B/RConn1 -- Line/LConn2
  b/RConn1 -- Line4/RConn2

== system ieee30/Line 27-30-1 ==
  Line{,1..4} (5 alike) : powerlib/Elements/Three-Phase PI Section Line  LConnTagsString=a|b|c  RConnTagsString=A|B|C  Frequency=60  Resistances=[rt ro] /100  Inductances=[ lt lo] /100  Capacitances=[ct co]/100  Length=20
      settings: SourceProductName=Simscape Power Systems
  A : PMIOPort  Port=1  Side=Left
  B : PMIOPort  Port=2  Side=Left
  C : PMIOPort  Port=3  Side=Left
  a : PMIOPort  Port=4  Side=Right
  b : PMIOPort  Port=5  Side=Right
  c : PMIOPort  Port=6  Side=Right
  connections:
  Line3/RConn3 -- Line4/LConn3
  Line/RConn3 -- Line1/LConn3
  Line2/RConn3 -- Line3/LConn3
  Line2/RConn1 -- Line3/LConn1
  Line1/RConn3 -- Line2/LConn3
  Line/RConn2 -- Line1/LConn2
  Line2/RConn2 -- Line3/LConn2
  Line1/RConn1 -- Line2/LConn1
  Line3/RConn1 -- Line4/LConn1
  Line3/RConn2 -- Line4/LConn2
  Line1/RConn2 -- Line2/LConn2
  Line/RConn1 -- Line1/LConn1
  C/RConn1 -- Line/LConn3
  Line/LConn1 -- A/RConn1
  c/RConn1 -- Line4/RConn3
  a/RConn1 -- Line4/RConn1
  B/RConn1 -- Line/LConn2
  b/RConn1 -- Line4/RConn2

== system ieee30/Line 27-30-2 ==
  Line{,1..4} (5 alike) : powerlib/Elements/Three-Phase PI Section Line  LConnTagsString=a|b|c  RConnTagsString=A|B|C  Frequency=60  Resistances=[rt ro] /100  Inductances=[ lt lo] /100  Capacitances=[ct co]/100  Length=20
      settings: SourceProductName=Simscape Power Systems
  A : PMIOPort  Port=1  Side=Left
  B : PMIOPort  Port=2  Side=Left
  C : PMIOPort  Port=3  Side=Left
  a : PMIOPort  Port=4  Side=Right
  b : PMIOPort  Port=5  Side=Right
  c : PMIOPort  Port=6  Side=Right
  connections:
  Line3/RConn3 -- Line4/LConn3
  Line/RConn3 -- Line1/LConn3
  Line2/RConn3 -- Line3/LConn3
  Line2/RConn1 -- Line3/LConn1
  Line1/RConn3 -- Line2/LConn3
  Line/RConn2 -- Line1/LConn2
  Line2/RConn2 -- Line3/LConn2
  Line1/RConn1 -- Line2/LConn1
  Line3/RConn1 -- Line4/LConn1
  Line3/RConn2 -- Line4/LConn2
  Line1/RConn2 -- Line2/LConn2
  Line/RConn1 -- Line1/LConn1
  C/RConn1 -- Line/LConn3
  Line/LConn1 -- A/RConn1
  c/RConn1 -- Line4/RConn3
  a/RConn1 -- Line4/RConn1
  B/RConn1 -- Line/LConn2
  b/RConn1 -- Line4/RConn2

== system ieee30/Line 29-30-1 ==
  Line{,1..4} (5 alike) : powerlib/Elements/Three-Phase PI Section Line  LConnTagsString=a|b|c  RConnTagsString=A|B|C  Frequency=60  Resistances=[rt ro] /100  Inductances=[ lt lo] /100  Capacitances=[ct co]/100  Length=20
      settings: SourceProductName=Simscape Power Systems
  A : PMIOPort  Port=1  Side=Left
  B : PMIOPort  Port=2  Side=Left
  C : PMIOPort  Port=3  Side=Left
  a : PMIOPort  Port=4  Side=Right
  b : PMIOPort  Port=5  Side=Right
  c : PMIOPort  Port=6  Side=Right
  connections:
  Line3/RConn3 -- Line4/LConn3
  Line/RConn3 -- Line1/LConn3
  Line2/RConn3 -- Line3/LConn3
  Line2/RConn1 -- Line3/LConn1
  Line1/RConn3 -- Line2/LConn3
  Line/RConn2 -- Line1/LConn2
  Line2/RConn2 -- Line3/LConn2
  Line1/RConn1 -- Line2/LConn1
  Line3/RConn1 -- Line4/LConn1
  Line3/RConn2 -- Line4/LConn2
  Line1/RConn2 -- Line2/LConn2
  Line/RConn1 -- Line1/LConn1
  C/RConn1 -- Line/LConn3
  Line/LConn1 -- A/RConn1
  c/RConn1 -- Line4/RConn3
  a/RConn1 -- Line4/RConn1
  B/RConn1 -- Line/LConn2
  b/RConn1 -- Line4/RConn2

== system ieee30/Line 29-30-2 ==
  Line{,1..4} (5 alike) : powerlib/Elements/Three-Phase PI Section Line  LConnTagsString=a|b|c  RConnTagsString=A|B|C  Frequency=60  Resistances=[rt ro] /100  Inductances=[ lt lo] /100  Capacitances=[ct co]/100  Length=20
      settings: SourceProductName=Simscape Power Systems
  A : PMIOPort  Port=1  Side=Left
  B : PMIOPort  Port=2  Side=Left
  C : PMIOPort  Port=3  Side=Left
  a : PMIOPort  Port=4  Side=Right
  b : PMIOPort  Port=5  Side=Right
  c : PMIOPort  Port=6  Side=Right
  connections:
  Line3/RConn3 -- Line4/LConn3
  Line/RConn3 -- Line1/LConn3
  Line2/RConn3 -- Line3/LConn3
  Line2/RConn1 -- Line3/LConn1
  Line1/RConn3 -- Line2/LConn3
  Line/RConn2 -- Line1/LConn2
  Line2/RConn2 -- Line3/LConn2
  Line1/RConn1 -- Line2/LConn1
  Line3/RConn1 -- Line4/LConn1
  Line3/RConn2 -- Line4/LConn2
  Line1/RConn2 -- Line2/LConn2
  Line/RConn1 -- Line1/LConn1
  C/RConn1 -- Line/LConn3
  Line/LConn1 -- A/RConn1
  c/RConn1 -- Line4/RConn3
  a/RConn1 -- Line4/RConn1
  B/RConn1 -- Line/LConn2
  b/RConn1 -- Line4/RConn2

== system ieee30/Line 3-4-1 ==
  Line{,1..4} (5 alike) : powerlib/Elements/Three-Phase PI Section Line  LConnTagsString=a|b|c  RConnTagsString=A|B|C  Frequency=60  Resistances=[rt ro] /100  Inductances=[ lt lo] /100  Capacitances=[ct co]/100  Length=20
      settings: SourceProductName=Simscape Power Systems
  A : PMIOPort  Port=1  Side=Left
  B : PMIOPort  Port=2  Side=Left
  C : PMIOPort  Port=3  Side=Left
  a : PMIOPort  Port=4  Side=Right
  b : PMIOPort  Port=5  Side=Right
  c : PMIOPort  Port=6  Side=Right
  connections:
  Line3/RConn3 -- Line4/LConn3
  Line/RConn3 -- Line1/LConn3
  Line2/RConn3 -- Line3/LConn3
  Line2/RConn1 -- Line3/LConn1
  Line1/RConn3 -- Line2/LConn3
  Line/RConn2 -- Line1/LConn2
  Line2/RConn2 -- Line3/LConn2
  Line1/RConn1 -- Line2/LConn1
  Line3/RConn1 -- Line4/LConn1
  Line3/RConn2 -- Line4/LConn2
  Line1/RConn2 -- Line2/LConn2
  Line/RConn1 -- Line1/LConn1
  C/RConn1 -- Line/LConn3
  Line/LConn1 -- A/RConn1
  c/RConn1 -- Line4/RConn3
  a/RConn1 -- Line4/RConn1
  B/RConn1 -- Line/LConn2
  b/RConn1 -- Line4/RConn2

== system ieee30/Line 3-4-2 ==
  Line{,1..4} (5 alike) : powerlib/Elements/Three-Phase PI Section Line  LConnTagsString=a|b|c  RConnTagsString=A|B|C  Frequency=60  Resistances=[rt ro] /100  Inductances=[ lt lo] /100  Capacitances=[ct co]/100  Length=20
      settings: SourceProductName=Simscape Power Systems
  A : PMIOPort  Port=1  Side=Left
  B : PMIOPort  Port=2  Side=Left
  C : PMIOPort  Port=3  Side=Left
  a : PMIOPort  Port=4  Side=Right
  b : PMIOPort  Port=5  Side=Right
  c : PMIOPort  Port=6  Side=Right
  connections:
  Line3/RConn3 -- Line4/LConn3
  Line/RConn3 -- Line1/LConn3
  Line2/RConn3 -- Line3/LConn3
  Line2/RConn1 -- Line3/LConn1
  Line1/RConn3 -- Line2/LConn3
  Line/RConn2 -- Line1/LConn2
  Line2/RConn2 -- Line3/LConn2
  Line1/RConn1 -- Line2/LConn1
  Line3/RConn1 -- Line4/LConn1
  Line3/RConn2 -- Line4/LConn2
  Line1/RConn2 -- Line2/LConn2
  Line/RConn1 -- Line1/LConn1
  C/RConn1 -- Line/LConn3
  Line/LConn1 -- A/RConn1
  c/RConn1 -- Line4/RConn3
  a/RConn1 -- Line4/RConn1
  B/RConn1 -- Line/LConn2
  b/RConn1 -- Line4/RConn2

== system ieee30/Line 4-6-1 ==
  Line{,1..4} (5 alike) : powerlib/Elements/Three-Phase PI Section Line  LConnTagsString=a|b|c  RConnTagsString=A|B|C  Frequency=60  Resistances=[rt ro] /100  Inductances=[ lt lo] /100  Capacitances=[ct co]/100  Length=20
      settings: SourceProductName=Simscape Power Systems
  A : PMIOPort  Port=1  Side=Left
  B : PMIOPort  Port=2  Side=Left
  C : PMIOPort  Port=3  Side=Left
  a : PMIOPort  Port=4  Side=Right
  b : PMIOPort  Port=5  Side=Right
  c : PMIOPort  Port=6  Side=Right
  connections:
  Line3/RConn3 -- Line4/LConn3
  Line/RConn3 -- Line1/LConn3
  Line2/RConn3 -- Line3/LConn3
  Line2/RConn1 -- Line3/LConn1
  Line1/RConn3 -- Line2/LConn3
  Line/RConn2 -- Line1/LConn2
  Line2/RConn2 -- Line3/LConn2
  Line1/RConn1 -- Line2/LConn1
  Line3/RConn1 -- Line4/LConn1
  Line3/RConn2 -- Line4/LConn2
  Line1/RConn2 -- Line2/LConn2
  Line/RConn1 -- Line1/LConn1
  C/RConn1 -- Line/LConn3
  Line/LConn1 -- A/RConn1
  c/RConn1 -- Line4/RConn3
  a/RConn1 -- Line4/RConn1
  B/RConn1 -- Line/LConn2
  b/RConn1 -- Line4/RConn2

== system ieee30/Line 4-6-2 ==
  Line{,1..4} (5 alike) : powerlib/Elements/Three-Phase PI Section Line  LConnTagsString=a|b|c  RConnTagsString=A|B|C  Frequency=60  Resistances=[rt ro] /100  Inductances=[ lt lo] /100  Capacitances=[ct co]/100  Length=20
      settings: SourceProductName=Simscape Power Systems
  A : PMIOPort  Port=1  Side=Left
  B : PMIOPort  Port=2  Side=Left
  C : PMIOPort  Port=3  Side=Left
  a : PMIOPort  Port=4  Side=Right
  b : PMIOPort  Port=5  Side=Right
  c : PMIOPort  Port=6  Side=Right
  connections:
  Line3/RConn3 -- Line4/LConn3
  Line/RConn3 -- Line1/LConn3
  Line2/RConn3 -- Line3/LConn3
  Line2/RConn1 -- Line3/LConn1
  Line1/RConn3 -- Line2/LConn3
  Line/RConn2 -- Line1/LConn2
  Line2/RConn2 -- Line3/LConn2
  Line1/RConn1 -- Line2/LConn1
  Line3/RConn1 -- Line4/LConn1
  Line3/RConn2 -- Line4/LConn2
  Line1/RConn2 -- Line2/LConn2
  Line/RConn1 -- Line1/LConn1
  C/RConn1 -- Line/LConn3
  Line/LConn1 -- A/RConn1
  c/RConn1 -- Line4/RConn3
  a/RConn1 -- Line4/RConn1
  B/RConn1 -- Line/LConn2
  b/RConn1 -- Line4/RConn2

== system ieee30/Line 5-7-1 ==
  Line{,1..4} (5 alike) : powerlib/Elements/Three-Phase PI Section Line  LConnTagsString=a|b|c  RConnTagsString=A|B|C  Frequency=60  Resistances=[rt ro] /100  Inductances=[ lt lo] /100  Capacitances=[ct co]/100  Length=20
      settings: SourceProductName=Simscape Power Systems
  A : PMIOPort  Port=1  Side=Left
  B : PMIOPort  Port=2  Side=Left
  C : PMIOPort  Port=3  Side=Left
  a : PMIOPort  Port=4  Side=Right
  b : PMIOPort  Port=5  Side=Right
  c : PMIOPort  Port=6  Side=Right
  connections:
  Line3/RConn3 -- Line4/LConn3
  Line/RConn3 -- Line1/LConn3
  Line2/RConn3 -- Line3/LConn3
  Line2/RConn1 -- Line3/LConn1
  Line1/RConn3 -- Line2/LConn3
  Line/RConn2 -- Line1/LConn2
  Line2/RConn2 -- Line3/LConn2
  Line1/RConn1 -- Line2/LConn1
  Line3/RConn1 -- Line4/LConn1
  Line3/RConn2 -- Line4/LConn2
  Line1/RConn2 -- Line2/LConn2
  Line/RConn1 -- Line1/LConn1
  C/RConn1 -- Line/LConn3
  Line/LConn1 -- A/RConn1
  c/RConn1 -- Line4/RConn3
  a/RConn1 -- Line4/RConn1
  B/RConn1 -- Line/LConn2
  b/RConn1 -- Line4/RConn2

== system ieee30/Line 5-7-2 ==
  Line{,1..4} (5 alike) : powerlib/Elements/Three-Phase PI Section Line  LConnTagsString=a|b|c  RConnTagsString=A|B|C  Frequency=60  Resistances=[rt ro] /100  Inductances=[ lt lo] /100  Capacitances=[ct co]/100  Length=20
      settings: SourceProductName=Simscape Power Systems
  A : PMIOPort  Port=1  Side=Left
  B : PMIOPort  Port=2  Side=Left
  C : PMIOPort  Port=3  Side=Left
  a : PMIOPort  Port=4  Side=Right
  b : PMIOPort  Port=5  Side=Right
  c : PMIOPort  Port=6  Side=Right
  connections:
  Line3/RConn3 -- Line4/LConn3
  Line/RConn3 -- Line1/LConn3
  Line2/RConn3 -- Line3/LConn3
  Line2/RConn1 -- Line3/LConn1
  Line1/RConn3 -- Line2/LConn3
  Line/RConn2 -- Line1/LConn2
  Line2/RConn2 -- Line3/LConn2
  Line1/RConn1 -- Line2/LConn1
  Line3/RConn1 -- Line4/LConn1
  Line3/RConn2 -- Line4/LConn2
  Line1/RConn2 -- Line2/LConn2
  Line/RConn1 -- Line1/LConn1
  C/RConn1 -- Line/LConn3
  Line/LConn1 -- A/RConn1
  c/RConn1 -- Line4/RConn3
  a/RConn1 -- Line4/RConn1
  B/RConn1 -- Line/LConn2
  b/RConn1 -- Line4/RConn2

== system ieee30/Line 6-28-1 ==
  Line{,1..4} (5 alike) : powerlib/Elements/Three-Phase PI Section Line  LConnTagsString=a|b|c  RConnTagsString=A|B|C  Frequency=60  Resistances=[rt ro] /100  Inductances=[ lt lo] /100  Capacitances=[ct co]/100  Length=20
      settings: SourceProductName=Simscape Power Systems
  A : PMIOPort  Port=1  Side=Left
  B : PMIOPort  Port=2  Side=Left
  C : PMIOPort  Port=3  Side=Left
  a : PMIOPort  Port=4  Side=Right
  b : PMIOPort  Port=5  Side=Right
  c : PMIOPort  Port=6  Side=Right
  connections:
  Line3/RConn3 -- Line4/LConn3
  Line/RConn3 -- Line1/LConn3
  Line2/RConn3 -- Line3/LConn3
  Line2/RConn1 -- Line3/LConn1
  Line1/RConn3 -- Line2/LConn3
  Line/RConn2 -- Line1/LConn2
  Line2/RConn2 -- Line3/LConn2
  Line1/RConn1 -- Line2/LConn1
  Line3/RConn1 -- Line4/LConn1
  Line3/RConn2 -- Line4/LConn2
  Line1/RConn2 -- Line2/LConn2
  Line/RConn1 -- Line1/LConn1
  C/RConn1 -- Line/LConn3
  Line/LConn1 -- A/RConn1
  c/RConn1 -- Line4/RConn3
  a/RConn1 -- Line4/RConn1
  B/RConn1 -- Line/LConn2
  b/RConn1 -- Line4/RConn2

== system ieee30/Line 6-28-2 ==
  Line{,1..4} (5 alike) : powerlib/Elements/Three-Phase PI Section Line  LConnTagsString=a|b|c  RConnTagsString=A|B|C  Frequency=60  Resistances=[rt ro] /100  Inductances=[ lt lo] /100  Capacitances=[ct co]/100  Length=20
      settings: SourceProductName=Simscape Power Systems
  A : PMIOPort  Port=1  Side=Left
  B : PMIOPort  Port=2  Side=Left
  C : PMIOPort  Port=3  Side=Left
  a : PMIOPort  Port=4  Side=Right
  b : PMIOPort  Port=5  Side=Right
  c : PMIOPort  Port=6  Side=Right
  connections:
  Line3/RConn3 -- Line4/LConn3
  Line/RConn3 -- Line1/LConn3
  Line2/RConn3 -- Line3/LConn3
  Line2/RConn1 -- Line3/LConn1
  Line1/RConn3 -- Line2/LConn3
  Line/RConn2 -- Line1/LConn2
  Line2/RConn2 -- Line3/LConn2
  Line1/RConn1 -- Line2/LConn1
  Line3/RConn1 -- Line4/LConn1
  Line3/RConn2 -- Line4/LConn2
  Line1/RConn2 -- Line2/LConn2
  Line/RConn1 -- Line1/LConn1
  C/RConn1 -- Line/LConn3
  Line/LConn1 -- A/RConn1
  c/RConn1 -- Line4/RConn3
  a/RConn1 -- Line4/RConn1
  B/RConn1 -- Line/LConn2
  b/RConn1 -- Line4/RConn2

== system ieee30/Line 6-7-1 ==
  Line{,1..4} (5 alike) : powerlib/Elements/Three-Phase PI Section Line  LConnTagsString=a|b|c  RConnTagsString=A|B|C  Frequency=60  Resistances=[rt ro] /100  Inductances=[ lt lo] /100  Capacitances=[ct co]/100  Length=20
      settings: SourceProductName=Simscape Power Systems
  A : PMIOPort  Port=1  Side=Left
  B : PMIOPort  Port=2  Side=Left
  C : PMIOPort  Port=3  Side=Left
  a : PMIOPort  Port=4  Side=Right
  b : PMIOPort  Port=5  Side=Right
  c : PMIOPort  Port=6  Side=Right
  connections:
  Line3/RConn3 -- Line4/LConn3
  Line/RConn3 -- Line1/LConn3
  Line2/RConn3 -- Line3/LConn3
  Line2/RConn1 -- Line3/LConn1
  Line1/RConn3 -- Line2/LConn3
  Line/RConn2 -- Line1/LConn2
  Line2/RConn2 -- Line3/LConn2
  Line1/RConn1 -- Line2/LConn1
  Line3/RConn1 -- Line4/LConn1
  Line3/RConn2 -- Line4/LConn2
  Line1/RConn2 -- Line2/LConn2
  Line/RConn1 -- Line1/LConn1
  C/RConn1 -- Line/LConn3
  Line/LConn1 -- A/RConn1
  c/RConn1 -- Line4/RConn3
  a/RConn1 -- Line4/RConn1
  B/RConn1 -- Line/LConn2
  b/RConn1 -- Line4/RConn2

== system ieee30/Line 6-7-2 ==
  Line{,1..4} (5 alike) : powerlib/Elements/Three-Phase PI Section Line  LConnTagsString=a|b|c  RConnTagsString=A|B|C  Frequency=60  Resistances=[rt ro] /100  Inductances=[ lt lo] /100  Capacitances=[ct co]/100  Length=20
      settings: SourceProductName=Simscape Power Systems
  A : PMIOPort  Port=1  Side=Left
  B : PMIOPort  Port=2  Side=Left
  C : PMIOPort  Port=3  Side=Left
  a : PMIOPort  Port=4  Side=Right
  b : PMIOPort  Port=5  Side=Right
  c : PMIOPort  Port=6  Side=Right
  connections:
  Line3/RConn3 -- Line4/LConn3
  Line/RConn3 -- Line1/LConn3
  Line2/RConn3 -- Line3/LConn3
  Line2/RConn1 -- Line3/LConn1
  Line1/RConn3 -- Line2/LConn3
  Line/RConn2 -- Line1/LConn2
  Line2/RConn2 -- Line3/LConn2
  Line1/RConn1 -- Line2/LConn1
  Line3/RConn1 -- Line4/LConn1
  Line3/RConn2 -- Line4/LConn2
  Line1/RConn2 -- Line2/LConn2
  Line/RConn1 -- Line1/LConn1
  C/RConn1 -- Line/LConn3
  Line/LConn1 -- A/RConn1
  c/RConn1 -- Line4/RConn3
  a/RConn1 -- Line4/RConn1
  B/RConn1 -- Line/LConn2
  b/RConn1 -- Line4/RConn2

== system ieee30/Line 6-8-1 ==
  Line{,1..4} (5 alike) : powerlib/Elements/Three-Phase PI Section Line  LConnTagsString=a|b|c  RConnTagsString=A|B|C  Frequency=60  Resistances=[rt ro] /100  Inductances=[ lt lo] /100  Capacitances=[ct co]/100  Length=20
      settings: SourceProductName=Simscape Power Systems
  A : PMIOPort  Port=1  Side=Left
  B : PMIOPort  Port=2  Side=Left
  C : PMIOPort  Port=3  Side=Left
  a : PMIOPort  Port=4  Side=Right
  b : PMIOPort  Port=5  Side=Right
  c : PMIOPort  Port=6  Side=Right
  connections:
  Line3/RConn3 -- Line4/LConn3
  Line/RConn3 -- Line1/LConn3
  Line2/RConn3 -- Line3/LConn3
  Line2/RConn1 -- Line3/LConn1
  Line1/RConn3 -- Line2/LConn3
  Line/RConn2 -- Line1/LConn2
  Line2/RConn2 -- Line3/LConn2
  Line1/RConn1 -- Line2/LConn1
  Line3/RConn1 -- Line4/LConn1
  Line3/RConn2 -- Line4/LConn2
  Line1/RConn2 -- Line2/LConn2
  Line/RConn1 -- Line1/LConn1
  C/RConn1 -- Line/LConn3
  Line/LConn1 -- A/RConn1
  c/RConn1 -- Line4/RConn3
  a/RConn1 -- Line4/RConn1
  B/RConn1 -- Line/LConn2
  b/RConn1 -- Line4/RConn2

== system ieee30/Line 6-8-2 ==
  Line{,1..4} (5 alike) : powerlib/Elements/Three-Phase PI Section Line  LConnTagsString=a|b|c  RConnTagsString=A|B|C  Frequency=60  Resistances=[rt ro] /100  Inductances=[ lt lo] /100  Capacitances=[ct co]/100  Length=20
      settings: SourceProductName=Simscape Power Systems
  A : PMIOPort  Port=1  Side=Left
  B : PMIOPort  Port=2  Side=Left
  C : PMIOPort  Port=3  Side=Left
  a : PMIOPort  Port=4  Side=Right
  b : PMIOPort  Port=5  Side=Right
  c : PMIOPort  Port=6  Side=Right
  connections:
  Line3/RConn3 -- Line4/LConn3
  Line/RConn3 -- Line1/LConn3
  Line2/RConn3 -- Line3/LConn3
  Line2/RConn1 -- Line3/LConn1
  Line1/RConn3 -- Line2/LConn3
  Line/RConn2 -- Line1/LConn2
  Line2/RConn2 -- Line3/LConn2
  Line1/RConn1 -- Line2/LConn1
  Line3/RConn1 -- Line4/LConn1
  Line3/RConn2 -- Line4/LConn2
  Line1/RConn2 -- Line2/LConn2
  Line/RConn1 -- Line1/LConn1
  C/RConn1 -- Line/LConn3
  Line/LConn1 -- A/RConn1
  c/RConn1 -- Line4/RConn3
  a/RConn1 -- Line4/RConn1
  B/RConn1 -- Line/LConn2
  b/RConn1 -- Line4/RConn2

== system ieee30/Line 8-28-1 ==
  Line{,1..4} (5 alike) : powerlib/Elements/Three-Phase PI Section Line  LConnTagsString=a|b|c  RConnTagsString=A|B|C  Frequency=60  Resistances=[rt ro] /100  Inductances=[ lt lo] /100  Capacitances=[ct co]/100  Length=20
      settings: SourceProductName=Simscape Power Systems
  A : PMIOPort  Port=1  Side=Left
  B : PMIOPort  Port=2  Side=Left
  C : PMIOPort  Port=3  Side=Left
  a : PMIOPort  Port=4  Side=Right
  b : PMIOPort  Port=5  Side=Right
  c : PMIOPort  Port=6  Side=Right
  connections:
  Line3/RConn3 -- Line4/LConn3
  Line/RConn3 -- Line1/LConn3
  Line2/RConn3 -- Line3/LConn3
  Line2/RConn1 -- Line3/LConn1
  Line1/RConn3 -- Line2/LConn3
  Line/RConn2 -- Line1/LConn2
  Line2/RConn2 -- Line3/LConn2
  Line1/RConn1 -- Line2/LConn1
  Line3/RConn1 -- Line4/LConn1
  Line3/RConn2 -- Line4/LConn2
  Line1/RConn2 -- Line2/LConn2
  Line/RConn1 -- Line1/LConn1
  C/RConn1 -- Line/LConn3
  Line/LConn1 -- A/RConn1
  c/RConn1 -- Line4/RConn3
  a/RConn1 -- Line4/RConn1
  B/RConn1 -- Line/LConn2
  b/RConn1 -- Line4/RConn2

== system ieee30/Line 8-28-2 ==
  Line{,1..4} (5 alike) : powerlib/Elements/Three-Phase PI Section Line  LConnTagsString=a|b|c  RConnTagsString=A|B|C  Frequency=60  Resistances=[rt ro] /100  Inductances=[ lt lo] /100  Capacitances=[ct co]/100  Length=20
      settings: SourceProductName=Simscape Power Systems
  A : PMIOPort  Port=1  Side=Left
  B : PMIOPort  Port=2  Side=Left
  C : PMIOPort  Port=3  Side=Left
  a : PMIOPort  Port=4  Side=Right
  b : PMIOPort  Port=5  Side=Right
  c : PMIOPort  Port=6  Side=Right
  connections:
  Line3/RConn3 -- Line4/LConn3
  Line/RConn3 -- Line1/LConn3
  Line2/RConn3 -- Line3/LConn3
  Line2/RConn1 -- Line3/LConn1
  Line1/RConn3 -- Line2/LConn3
  Line/RConn2 -- Line1/LConn2
  Line2/RConn2 -- Line3/LConn2
  Line1/RConn1 -- Line2/LConn1
  Line3/RConn1 -- Line4/LConn1
  Line3/RConn2 -- Line4/LConn2
  Line1/RConn2 -- Line2/LConn2
  Line/RConn1 -- Line1/LConn1
  C/RConn1 -- Line/LConn3
  Line/LConn1 -- A/RConn1
  c/RConn1 -- Line4/RConn3
  a/RConn1 -- Line4/RConn1
  B/RConn1 -- Line/LConn2
  b/RConn1 -- Line4/RConn2
